simulink model "sssClutch"  (Simulink 8.3)
settings: Solver=ode3  StartTime=0.0  StopTime=150  FixedStep=0.05  RelTol=1e-3
settings Model: Creator=Administrator  LastModifiedBy=Administrator
settings DataIOCC: SignalLoggingSaveFormat=Dataset
settings DebuggingCC: UnderspecifiedInitializationDetection=Simplified  StateNameClashWarn=none
settings GRTTargetCC: CombineOutputUpdateFcns=on  GRTInterface=off

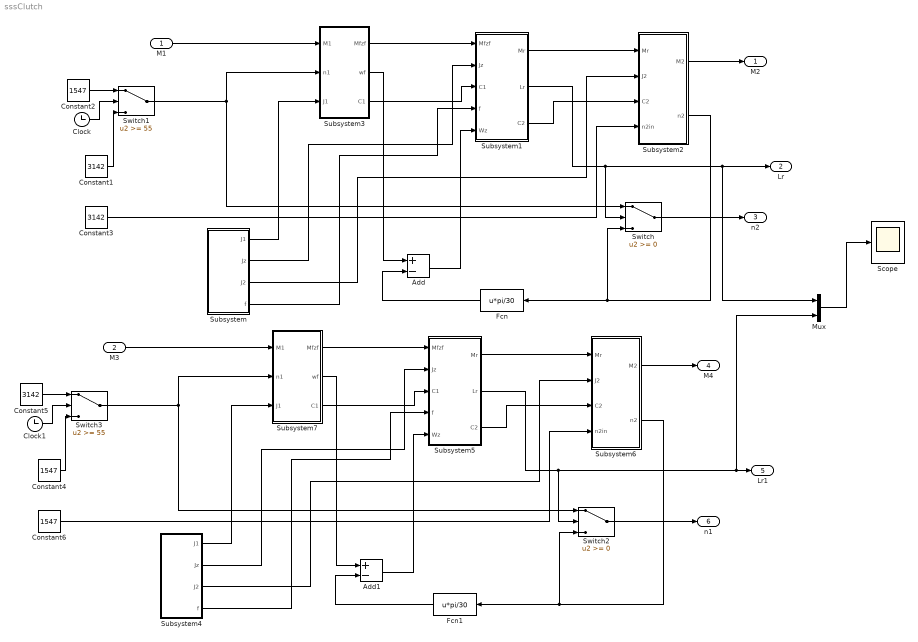
== system sssClutch ==
  M1 : Inport
  M3 : Inport  Port=2
  Add : Sum  Inputs=+-
  Add1 : Sum  Inputs=+-
  Clock : Clock
  Clock1 : Clock
  Constant1 : Constant  Value=3142
  Constant2 : Constant  Value=1547
  Constant3 : Constant  Value=3142
  Constant4 : Constant  Value=1547
  Constant5 : Constant  Value=3142
  Constant6 : Constant  Value=1547
  Fcn : Fcn  Expr=u*pi/30
  Fcn1 : Fcn  Expr=u*pi/30
  Mux : Mux  Inputs=2
  Scope : Scope
      settings: TimeRange=100  YMin=0  YMax=15
  Subsystem : Subsystem
  Subsystem1 : Subsystem
  Subsystem2 : Subsystem
  Subsystem3 : Subsystem
  Subsystem4 : Subsystem
  Subsystem5 : Subsystem
  Subsystem6 : Subsystem
  Subsystem7 : Subsystem
  Switch : Switch
  Switch1 : Switch  Threshold=55
  Switch2 : Switch
  Switch3 : Switch  Threshold=55
  M2 : Outport
  Lr : Outport  Port=2
  n2 : Outport  Port=3
  M4 : Outport  Port=4
  Lr1 : Outport  Port=5
  n1 : Outport  Port=6
  wires:
  Fcn/1 -> Add/2
  Switch/1 -> n2/1
  M1/1 -> Subsystem3/1(M1)
  Subsystem/1(J1) -> Subsystem3/3(J1)
  Subsystem/2(Jz) -> Subsystem1/2(Jz)
  Subsystem3/1(Mfzf) -> Subsystem1/1(Mfzf)
  Subsystem3/3(C1) -> Subsystem1/3(C1)
  Subsystem1/1(Mr) -> Subsystem2/1(Mr)
  Subsystem1/3(C2) -> Subsystem2/3(C2)
  Subsystem3/2(wf) -> Add/1
  Subsystem/3(J2) -> Subsystem2/2(J2)
  Subsystem2/1(M2) -> M2/1
  Subsystem/4(f) -> Subsystem1/4(f)
  Constant3/1 -> Subsystem2/4(n2in)
  Add/1 -> Subsystem1/5(Wz)
  Subsystem2/2(n2) -> Fcn/1, Switch/3
  Switch1/1 -> Subsystem3/2(n1), Switch/1
  Subsystem1/2(Lr) -> Switch/2, Mux/1, Lr/1
  Clock/1 -> Switch1/2
  Constant1/1 -> Switch1/3
  Constant2/1 -> Switch1/1
  Fcn1/1 -> Add1/2
  Switch2/1 -> n1/1
  M3/1 -> Subsystem7/1(M1)
  Subsystem4/1(J1) -> Subsystem7/3(J1)
  Subsystem4/2(Jz) -> Subsystem5/2(Jz)
  Subsystem7/1(Mfzf) -> Subsystem5/1(Mfzf)
  Subsystem7/3(C1) -> Subsystem5/3(C1)
  Subsystem5/1(Mr) -> Subsystem6/1(Mr)
  Subsystem5/3(C2) -> Subsystem6/3(C2)
  Subsystem7/2(wf) -> Add1/1
  Subsystem4/3(J2) -> Subsystem6/2(J2)
  Subsystem6/1(M2) -> M4/1
  Subsystem4/4(f) -> Subsystem5/4(f)
  Constant6/1 -> Subsystem6/4(n2in)
  Add1/1 -> Subsystem5/5(Wz)
  Subsystem6/2(n2) -> Fcn1/1, Switch2/3
  Switch3/1 -> Subsystem7/2(n1), Switch2/1
  Subsystem5/2(Lr) -> Switch2/2, Mux/2, Lr1/1
  Clock1/1 -> Switch3/2
  Constant4/1 -> Switch3/3
  Constant5/1 -> Switch3/1
  Mux/1 -> Scope/1

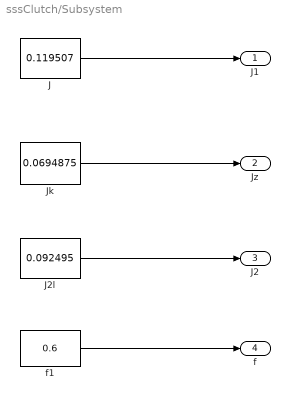
== system sssClutch/Subsystem ==
  J : Constant  Value=0.119507
  J2l : Constant  Value=0.092495
  Jk : Constant  Value=0.0694875
  f1 : Constant  Value=0.6
  J1 : Outport
  Jz : Outport  Port=2
  J2 : Outport  Port=3
  f : Outport  Port=4
  wires:
  J/1 -> J1/1
  Jk/1 -> Jz/1
  J2l/1 -> J2/1
  f1/1 -> f/1

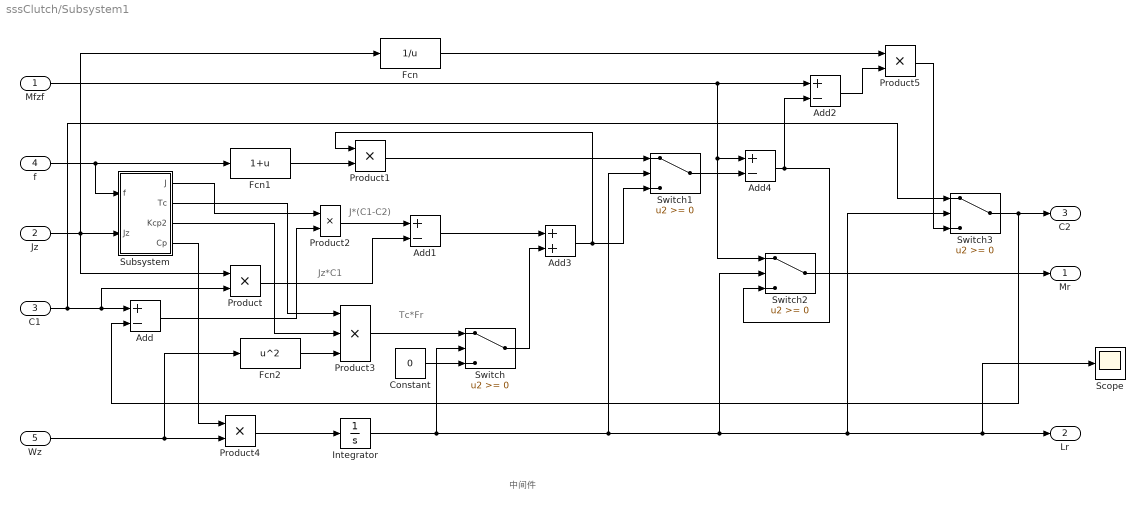
== system sssClutch/Subsystem1 ==
  note: Tc*Fr
  note: Jz*C1
  note: J*(C1-C2)
  note: 中间件
  Mfzf : Inport
  Jz : Inport  Port=2
  C1 : Inport  Port=3
  f : Inport  Port=4
  Wz : Inport  Port=5
  Add{,1..2,4} (4 alike) : Sum  Inputs=+-
  Add3 : Sum
  Constant : Constant  Value=0
  Fcn : Fcn  Expr=1/u
  Fcn1 : Fcn  Expr=1+u
  Fcn2 : Fcn  Expr=u^2
  Integrator : Integrator  InitialCondition=15  LimitOutput=on  UpperSaturationLimit=15  LowerSaturationLimit=0
  Product{,1..2,4..5} (5 alike) : Product
  Product3 : Product  Inputs=3
  Scope : Scope
  Subsystem : Subsystem
  Switch{,1..3} (4 alike) : Switch
  Mr : Outport
  Lr : Outport  Port=2
  C2 : Outport  Port=3
  wires:
  C1/1 -> Switch3/1, Product/2, Add/1
  f/1 -> Subsystem/1(f), Fcn1/1
  Fcn1/1 -> Product1/2
  Product1/1 -> Switch1/1
  Switch1/1 -> Add4/2
  Mfzf/1 -> Add2/1, Add4/1, Switch2/1
  Add2/1 -> Product5/2
  Fcn/1 -> Product5/1
  Switch2/1 -> Mr/1
  Jz/1 -> Product/1, Subsystem/2(Jz), Fcn/1
  Wz/1 -> Fcn2/1, Product4/2
  Fcn2/1 -> Product3/3
  Product4/1 -> Integrator/1
  Integrator/1 -> Scope/1, Lr/1, Switch3/2, Switch2/2, Switch1/2, Switch/2
  Product3/1 -> Switch/1
  Constant/1 -> Switch/3
  Add1/1 -> Add3/1
  Switch/1 -> Add3/2
  Add3/1 -> Product1/1, Switch1/3
  Product/1 -> Add1/2
  Product2/1 -> Add1/1
  Add/1 -> Product2/2
  Subsystem/4(Cp) -> Product4/1
  Subsystem/3(Kcp2) -> Product3/2
  Subsystem/1(J) -> Product2/1
  Subsystem/2(Tc) -> Product3/1
  Product5/1 -> Switch3/3
  Add4/1 -> Add2/2, Switch2/3
  Switch3/1 -> Add/2, C2/1

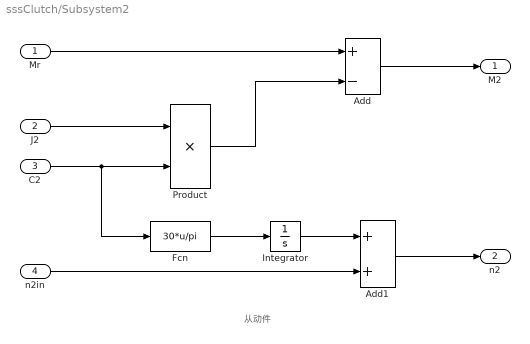
== system sssClutch/Subsystem2 ==
  note: 从动件
  Mr : Inport
  J2 : Inport  Port=2
  C2 : Inport  Port=3
  n2in : Inport  Port=4
  Add : Sum  Inputs=+-
  Add1 : Sum
  Fcn : Fcn  Expr=30*u/pi
  Integrator : Integrator
  Product : Product
  M2 : Outport
  n2 : Outport  Port=2
  wires:
  Mr/1 -> Add/1
  Add/1 -> M2/1
  J2/1 -> Product/1
  C2/1 -> Fcn/1, Product/2
  Fcn/1 -> Integrator/1
  Integrator/1 -> Add1/1
  n2in/1 -> Add1/2
  Add1/1 -> n2/1
  Product/1 -> Add/2

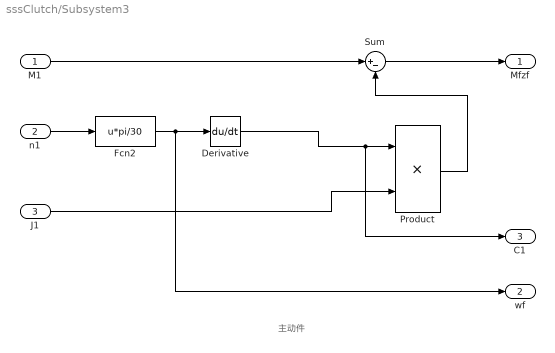
== system sssClutch/Subsystem3 ==
  note: 主动件
  M1 : Inport
  n1 : Inport  Port=2
  J1 : Inport  Port=3
  Derivative : Derivative
  Fcn2 : Fcn  Expr=u*pi/30
  Product : Product
  Sum : Sum  Inputs=|+-
  Mfzf : Outport
  wf : Outport  Port=2
  C1 : Outport  Port=3
  wires:
  n1/1 -> Fcn2/1
  Fcn2/1 -> wf/1, Derivative/1
  M1/1 -> Sum/1
  J1/1 -> Product/2
  Derivative/1 -> C1/1, Product/1
  Product/1 -> Sum/2
  Sum/1 -> Mfzf/1

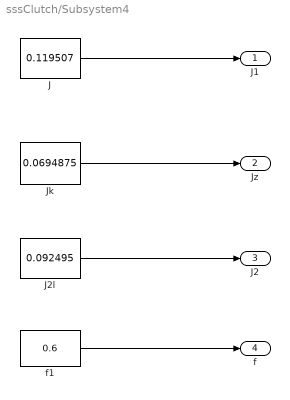
== system sssClutch/Subsystem4 ==
  J : Constant  Value=0.119507
  J2l : Constant  Value=0.092495
  Jk : Constant  Value=0.0694875
  f1 : Constant  Value=0.6
  J1 : Outport
  Jz : Outport  Port=2
  J2 : Outport  Port=3
  f : Outport  Port=4
  wires:
  J/1 -> J1/1
  Jk/1 -> Jz/1
  J2l/1 -> J2/1
  f1/1 -> f/1

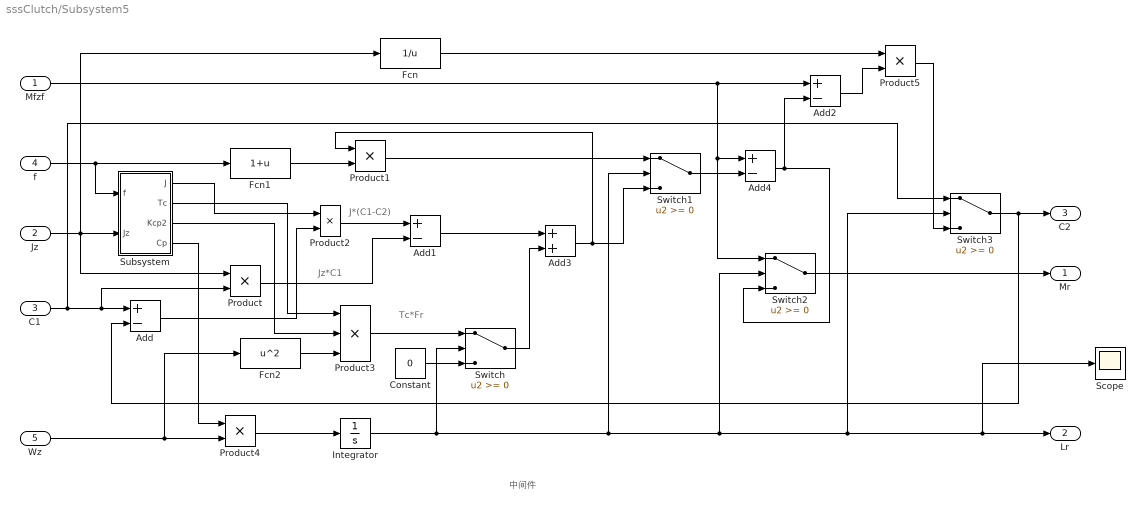
== system sssClutch/Subsystem5 ==
  note: Tc*Fr
  note: Jz*C1
  note: J*(C1-C2)
  note: 中间件
  Mfzf : Inport
  Jz : Inport  Port=2
  C1 : Inport  Port=3
  f : Inport  Port=4
  Wz : Inport  Port=5
  Add{,1..2,4} (4 alike) : Sum  Inputs=+-
  Add3 : Sum
  Constant : Constant  Value=0
  Fcn : Fcn  Expr=1/u
  Fcn1 : Fcn  Expr=1+u
  Fcn2 : Fcn  Expr=u^2
  Integrator : Integrator  LimitOutput=on  UpperSaturationLimit=15  LowerSaturationLimit=0
  Product{,1..2,4..5} (5 alike) : Product
  Product3 : Product  Inputs=3
  Scope : Scope
  Subsystem : Subsystem
  Switch{,1..3} (4 alike) : Switch
  Mr : Outport
  Lr : Outport  Port=2
  C2 : Outport  Port=3
  wires:
  C1/1 -> Switch3/1, Product/2, Add/1
  f/1 -> Subsystem/1(f), Fcn1/1
  Fcn1/1 -> Product1/2
  Product1/1 -> Switch1/1
  Switch1/1 -> Add4/2
  Mfzf/1 -> Add2/1, Add4/1, Switch2/1
  Add2/1 -> Product5/2
  Fcn/1 -> Product5/1
  Switch2/1 -> Mr/1
  Jz/1 -> Product/1, Subsystem/2(Jz), Fcn/1
  Wz/1 -> Fcn2/1, Product4/2
  Fcn2/1 -> Product3/3
  Product4/1 -> Integrator/1
  Integrator/1 -> Scope/1, Lr/1, Switch3/2, Switch2/2, Switch1/2, Switch/2
  Product3/1 -> Switch/1
  Constant/1 -> Switch/3
  Add1/1 -> Add3/1
  Switch/1 -> Add3/2
  Add3/1 -> Product1/1, Switch1/3
  Product/1 -> Add1/2
  Product2/1 -> Add1/1
  Add/1 -> Product2/2
  Subsystem/4(Cp) -> Product4/1
  Subsystem/3(Kcp2) -> Product3/2
  Subsystem/1(J) -> Product2/1
  Subsystem/2(Tc) -> Product3/1
  Product5/1 -> Switch3/3
  Add4/1 -> Add2/2, Switch2/3
  Switch3/1 -> Add/2, C2/1

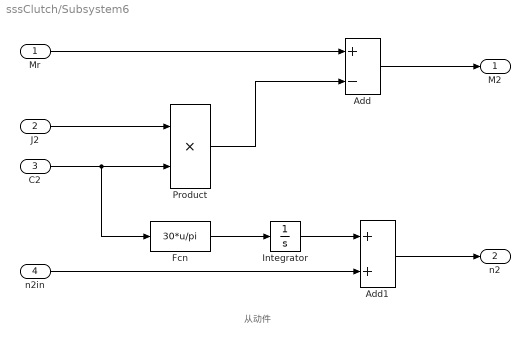
== system sssClutch/Subsystem6 ==
  note: 从动件
  Mr : Inport
  J2 : Inport  Port=2
  C2 : Inport  Port=3
  n2in : Inport  Port=4
  Add : Sum  Inputs=+-
  Add1 : Sum
  Fcn : Fcn  Expr=30*u/pi
  Integrator : Integrator
  Product : Product
  M2 : Outport
  n2 : Outport  Port=2
  wires:
  Mr/1 -> Add/1
  Add/1 -> M2/1
  J2/1 -> Product/1
  C2/1 -> Fcn/1, Product/2
  Fcn/1 -> Integrator/1
  Integrator/1 -> Add1/1
  n2in/1 -> Add1/2
  Add1/1 -> n2/1
  Product/1 -> Add/2

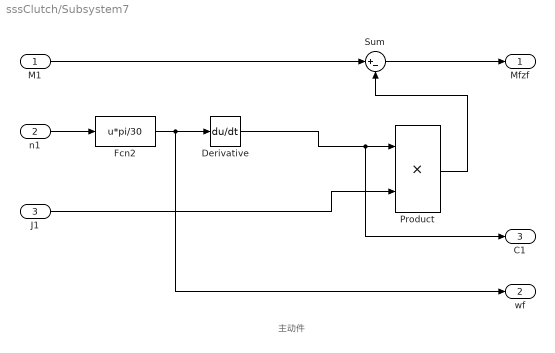
== system sssClutch/Subsystem7 ==
  note: 主动件
  M1 : Inport
  n1 : Inport  Port=2
  J1 : Inport  Port=3
  Derivative : Derivative
  Fcn2 : Fcn  Expr=u*pi/30
  Product : Product
  Sum : Sum  Inputs=|+-
  Mfzf : Outport
  wf : Outport  Port=2
  C1 : Outport  Port=3
  wires:
  n1/1 -> Fcn2/1
  Fcn2/1 -> wf/1, Derivative/1
  M1/1 -> Sum/1
  J1/1 -> Product/2
  Derivative/1 -> C1/1, Product/1
  Product/1 -> Sum/2
  Sum/1 -> Mfzf/1

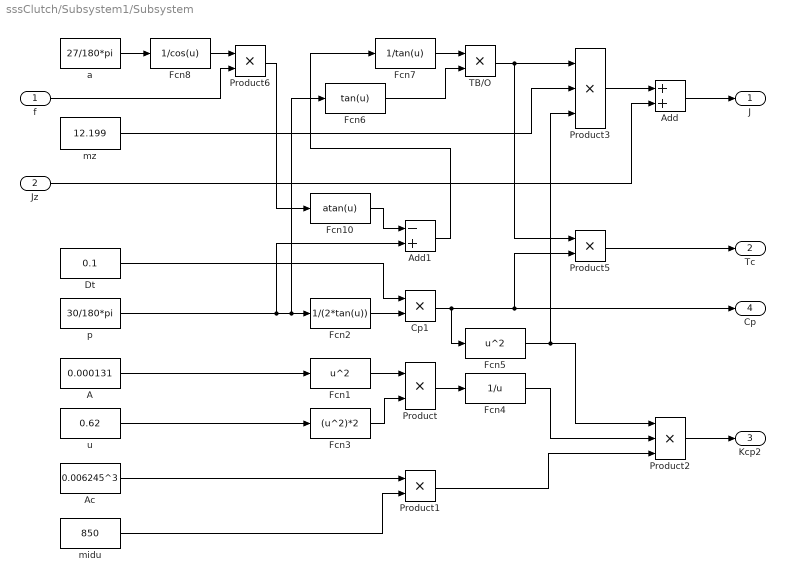
== system sssClutch/Subsystem1/Subsystem ==
  f : Inport
  Jz : Inport  Port=2
  A : Constant  Value=0.000131
  Ac : Constant  Value=0.006245^3
  Add : Sum
  Add1 : Sum  Inputs=-+
  Cp1 : Product  RndMeth=Zero
  Dt : Constant  Value=0.1
  Fcn1 : Fcn  Expr=u^2
  Fcn10 : Fcn  Expr=atan(u)
  Fcn2 : Fcn  Expr=1/(2*tan(u))
  Fcn3 : Fcn  Expr=(u^2)*2
  Fcn4 : Fcn  Expr=1/u
  Fcn5 : Fcn  Expr=u^2
  Fcn6 : Fcn  Expr=tan(u)
  Fcn7 : Fcn  Expr=1/tan(u)
  Fcn8 : Fcn  Expr=1/cos(u)
  Product{,1,5..6} (4 alike) : Product  RndMeth=Zero
  Product2 : Product  Inputs=3  RndMeth=Zero
  Product3 : Product  Inputs=3  RndMeth=Zero
  TB/O : Product  RndMeth=Zero
  a : Constant  Value=27/180*pi
  midu : Constant  Value=850
  mz : Constant  Value=12.199
  p : Constant  Value=30/180*pi
  u : Constant  Value=0.62
  J : Outport
  Tc : Outport  Port=2
  Kcp2 : Outport  Port=3
  Cp : Outport  Port=4
  wires:
  p/1 -> Fcn2/1, Fcn6/1, Add1/2
  Dt/1 -> Cp1/1
  Fcn2/1 -> Cp1/2
  Cp1/1 -> Cp/1, Product5/2, Fcn5/1
  A/1 -> Fcn1/1
  u/1 -> Fcn3/1
  Fcn3/1 -> Product/2
  Fcn1/1 -> Product/1
  Product/1 -> Fcn4/1
  Ac/1 -> Product1/1
  midu/1 -> Product1/2
  Product1/1 -> Product2/3
  Product2/1 -> Kcp2/1
  Fcn4/1 -> Product2/2
  Fcn5/1 -> Product2/1, Product3/3
  a/1 -> Fcn8/1
  Product3/1 -> Add/1
  Jz/1 -> Add/2
  Add/1 -> J/1
  Fcn7/1 -> TB/O/1
  Fcn6/1 -> TB/O/2
  TB/O/1 -> Product3/1, Product5/1
  mz/1 -> Product3/2
  Product5/1 -> Tc/1
  Fcn8/1 -> Product6/1
  f/1 -> Product6/2
  Product6/1 -> Fcn10/1
  Fcn10/1 -> Add1/1
  Add1/1 -> Fcn7/1

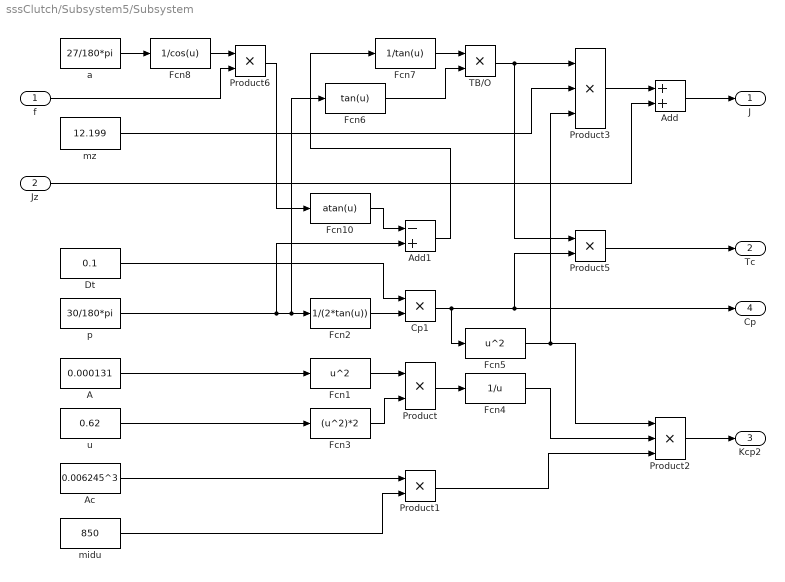
== system sssClutch/Subsystem5/Subsystem ==
  f : Inport
  Jz : Inport  Port=2
  A : Constant  Value=0.000131
  Ac : Constant  Value=0.006245^3
  Add : Sum
  Add1 : Sum  Inputs=-+
  Cp1 : Product  RndMeth=Zero
  Dt : Constant  Value=0.1
  Fcn1 : Fcn  Expr=u^2
  Fcn10 : Fcn  Expr=atan(u)
  Fcn2 : Fcn  Expr=1/(2*tan(u))
  Fcn3 : Fcn  Expr=(u^2)*2
  Fcn4 : Fcn  Expr=1/u
  Fcn5 : Fcn  Expr=u^2
  Fcn6 : Fcn  Expr=tan(u)
  Fcn7 : Fcn  Expr=1/tan(u)
  Fcn8 : Fcn  Expr=1/cos(u)
  Product{,1,5..6} (4 alike) : Product  RndMeth=Zero
  Product2 : Product  Inputs=3  RndMeth=Zero
  Product3 : Product  Inputs=3  RndMeth=Zero
  TB/O : Product  RndMeth=Zero
  a : Constant  Value=27/180*pi
  midu : Constant  Value=850
  mz : Constant  Value=12.199
  p : Constant  Value=30/180*pi
  u : Constant  Value=0.62
  J : Outport
  Tc : Outport  Port=2
  Kcp2 : Outport  Port=3
  Cp : Outport  Port=4
  wires:
  p/1 -> Fcn2/1, Fcn6/1, Add1/2
  Dt/1 -> Cp1/1
  Fcn2/1 -> Cp1/2
  Cp1/1 -> Cp/1, Product5/2, Fcn5/1
  A/1 -> Fcn1/1
  u/1 -> Fcn3/1
  Fcn3/1 -> Product/2
  Fcn1/1 -> Product/1
  Product/1 -> Fcn4/1
  Ac/1 -> Product1/1
  midu/1 -> Product1/2
  Product1/1 -> Product2/3
  Product2/1 -> Kcp2/1
  Fcn4/1 -> Product2/2
  Fcn5/1 -> Product2/1, Product3/3
  a/1 -> Fcn8/1
  Product3/1 -> Add/1
  Jz/1 -> Add/2
  Add/1 -> J/1
  Fcn7/1 -> TB/O/1
  Fcn6/1 -> TB/O/2
  TB/O/1 -> Product3/1, Product5/1
  mz/1 -> Product3/2
  Product5/1 -> Tc/1
  Fcn8/1 -> Product6/1
  f/1 -> Product6/2
  Product6/1 -> Fcn10/1
  Fcn10/1 -> Add1/1
  Add1/1 -> Fcn7/1
